simulink model "bsp_ev3_gyro_absdps"  (R2019a)
settings: Solver=FixedStepAuto  StartTime=0.0  StopTime=20  FixedStep=0.1  RelTol=1e-3  EnableMultiTasking=on
libraries: BrickPiSimSubLib_initreset x2, BrickPiSimSubLib_getsensor x1
settings Model: SimulationMode=external  Creator=uk008555  LastModifiedBy=uk008555
settings SolverCC: PositivePriorityOrder=on
settings OptimizationCC: EnhancedBackFolding=on  PassReuseOutputArgsAs=Individual arguments  MaxStackSize=64  OptimizeBlockOrder=speed  DifferentSizesBufferReuse=on  OptimizationCustomize=off
settings DebuggingCC: ParameterTunabilityLossMsg=error
settings HardwareCC: ProdBitPerPointer=32  ProdBitPerSizeT=32  ProdBitPerPtrDiffT=32  ProdLargestAtomicInteger=Long  ProdLargestAtomicFloat=Double  ProdWordSize=32  ProdLongLongMode=on  ProdHWDeviceType=ARM Compatible->ARM Cortex
settings SFSimCC: MATLABDynamicMemAlloc=off
settings RTWCC: SystemTargetFile=ert.tlc  HardwareBoard=Raspberry Pi  TLCOptions="-aInlineSetEventsForThisBaseRateFcn=TLC_FALSE -aSuppressMultiTaskScheduler=TLC_FALSE  -aRateBasedStepFcn=0"  TemplateMakefile=ert_default_tmf  GenerateReport=on  Toolchain=GNU GCC Raspberry Pi  BuildConfiguration=Faster Runs  IncludeHyperlinkInReport=on  LaunchReport=on  GenerateTraceInfo=on  GenerateTraceReport=on  GenerateTraceReportSl=on  GenerateTraceReportSf=on  GenerateTraceReportEml=on
settings CodeAppCC: ForceParamTrailComments=on  IgnoreCustomStorageClasses=off  OperatorAnnotations=on  SimulinkDataObjDesc=on  SFDataObjDesc=on  InsertBlockDesc=on
settings ERTTargetCC: SupportVariableSizeSignals=on

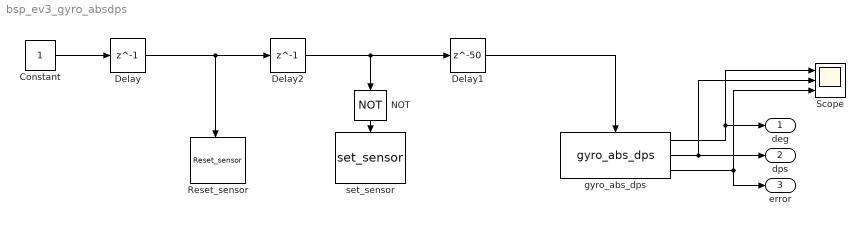
== system bsp_ev3_gyro_absdps ==
  Constant : Constant
  Delay : Delay  DelayLength=1
  Delay1 : Delay  DelayLength=50
  Delay2 : Delay  DelayLength=1
  NOT : Logic  Operator=NOT  IconShape=distinctive  AllPortsSameDT=off  OutDataTypeStr=boolean
  Reset_sensor : BrickPiSimSubLib_initreset/Reset_sensor  Port1_Val=off  Port2_Val=off  Port3_Val=on  Port4_Val=off
      settings: SourceProductName=Simulink Support Package for BrickPi
  Scope : Scope  NumInputPorts=3
  gyro_abs_dps : BrickPiSimSubLib_getsensor/gyro_abs_dps  Add_Val=1  Port_Val=3
      settings: SourceProductName=Simulink Support Package for BrickPi
  set_sensor : BrickPiSimSubLib_initreset/set_sensor  Add_Val=1  Type_Val=Ev3 ABS & DPS  Port_Val=3
      settings: SourceProductName=Simulink Support Package for BrickPi
  deg : Outport
  dps : Outport  Port=2
  error : Outport  Port=3
  wires:
  gyro_abs_dps/1 -> Scope/1, deg/1
  gyro_abs_dps/3 -> Scope/3, error/1
  Constant/1 -> Delay/1
  Delay/1 -> Delay2/1, Reset_sensor/Enable
  Delay1/1 -> gyro_abs_dps/Enable
  NOT/1 -> set_sensor/Enable
  gyro_abs_dps/2 -> Scope/2, dps/1
  Delay2/1 -> NOT/1, Delay1/1
